simulink model "PM_Motor_Ver2015"  (R2015a)
settings: Solver=VariableStepDiscrete  StartTime=0.0  StopTime=1  RelTol=1e-3
PreLoadFcn:
  | Ts=5e-6;
undefined symbols (not defined in the file): ctrl_sat, pos_Kp, Pos_Target, speed_Ki, speed_Kp, Speed_Target
libraries: powerlib x16, powerlib_extras x3, simulink x1, AC6DriveInternalModels x1
settings Model: ExtModeAutoUpdateStatusClock=off  Creator=batserve  LastModifiedBy=Savvas
settings DataIOCC: SignalLoggingSaveFormat=ModelDataLogs  SaveOutput=off  SignalLogging=off  SaveTime=off  SignalLoggingName=sigsOut
settings OptimizationCC: ExpressionDepthLimit=2147483647  InitFltsAndDblsToZero=on
settings DebuggingCC: SaveWithParameterizedLinksMsg=none  UnderspecifiedInitializationDetection=Classic  MergeDetectMultiDrivingBlocksExec=none  CheckExecutionContextPreStartOutputMsg=on  CheckExecutionContextRuntimeOutputMsg=on  SignalResolutionControl=TryResolveAllWithWarning  MultiTaskDSMMsg=warning  MultiTaskCondExecSysMsg=none  FcnCallInpInsideContextMsg=UseLocalSettings  StateNameClashWarn=warning
settings HardwareCC: TargetUnknown=on
settings GRTTargetCC: TargetFcnLib=ansi_tfl_tmw.mat  CombineOutputUpdateFcns=off  GRTInterface=on

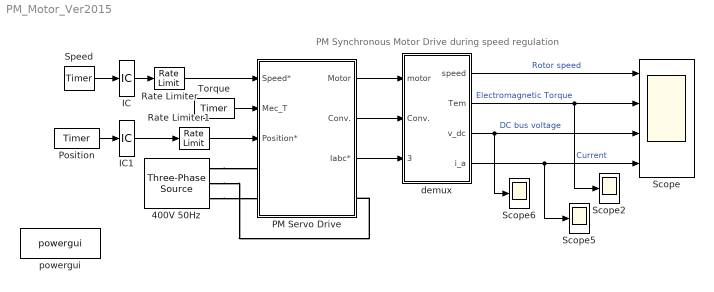
== system PM_Motor_Ver2015 ==
  note: PM Synchronous Motor Drive during speed regulation
  400V 50Hz : powerlib/Electrical Sources/Three-Phase Source  Voltage=400  PhaseAngle=0  Frequency=60  InternalConnection=Yg  SpecifyImpedance=off  Resistance=0.02  Inductance=0.05e-3  ShortCircuitLevel=100e6  BaseVoltage=25e3  XRratio=7  BusType=swing  Pref=0  Qref=0  Qmin=-inf  Qmax=inf
  IC : InitialCondition  Value=0
  IC1 : InitialCondition  Value=0
  PM Servo Drive : Subsystem
  Position : powerlib_extras/Control  Blocks/Timer  t=[0 1]  e=[1 1]*Pos_Target
  Rate Limiter : RateLimiter  RisingSlewLimit=600000  FallingSlewLimit=-600000  LinearizeAsGain=off
  Rate Limiter1 : RateLimiter  RisingSlewLimit=2000  FallingSlewLimit=-2000  SampleTimeMode=inherited  LinearizeAsGain=off
  Scope : Scope  NumInputPorts=4
      settings: TimeRange=0.5  YMin=-1500~-30~0~-60  YMax=1500~30~1000~60  SaveName=simout
  Scope2 : Scope
      settings: YMin=-15  YMax=25  SaveName=Torque
  Scope5 : Scope
      settings: TimeRange=0.06746987951807232  YMin=-30.19796761679877  YMax=24.82817507168159  SaveName=Current
  Scope6 : Scope
      settings: YMin=-1500  YMax=1500  SaveName=DC_voltage
  Speed : powerlib_extras/Control  Blocks/Timer  t=[0 1]  e=[1 1]*Speed_Target
  Torque : powerlib_extras/Control  Blocks/Timer  t=Mech_Load_Time  e=Mech_Load
  demux : Subsystem
  powergui : powerlib/powergui  Priority=2  SimulationMode=Discrete  SolverType=Tustin  SampleTime=Ts  frequency=60  SPID=off  DisableSnubberDevices=off  DisableRonSwitches=off  DisableVfSwitches=off  SwTol=0  DisplayEquations=off  Interpol=off  methode=off  Ts=0  FunctionMessages=off  echomessages=off  HookPort=off  EnableUseOfTLC=off  x0status=blocks  frequencyindice=60  Pbase=100e6  ErrMax=1e-4  Iterations=50  UnitsV=kV  UnitsW=MW  buscounter=0  RestoreLinks=warning  ResistiveCurrentMeasurement=off  Frange=[0:2:500]  Ylog=off  Xlog=on  ShowGrid=off  save=off  variable=ZData  structure=0  ZoomFFT=on  StartTime=0.0  cycles=1  DisplayStyle=1  fundamental=60  FreqAxis=off  MaxFrequency=1000  frequencyindicesteady=1  RmsSteady=1  display=off
  wires:
  Torque/1 -> PM Servo Drive/2(Mec_T)
  PM Servo Drive/1(Motor) -> demux/1(motor)
  PM Servo Drive/2(Conv.) -> demux/2(Conv.)
  PM Servo Drive/3(Iabc*) -> demux/3(Conv.2)
  demux/1(speed) -> Scope/1  "Rotor speed"
  demux/2(Tem) -> Scope/2, Scope2/1  "Electromagnetic Torque"
  demux/3(v_dc) -> Scope/3, Scope6/1  "DC bus voltage"
  demux/4(i_a) -> Scope/4, Scope5/1  "Current"
  Speed/1 -> IC/1
  Position/1 -> IC1/1
  Rate Limiter/1 -> PM Servo Drive/1(Speed*)
  Rate Limiter1/1 -> PM Servo Drive/3(Position*)
  IC/1 -> Rate Limiter/1
  IC1/1 -> Rate Limiter1/1
  connections:
  400V 50Hz/RConn1 -- PM Servo Drive/LConn1
  400V 50Hz/RConn2 -- PM Servo Drive/RConn1
  400V 50Hz/RConn3 -- PM Servo Drive/LConn2

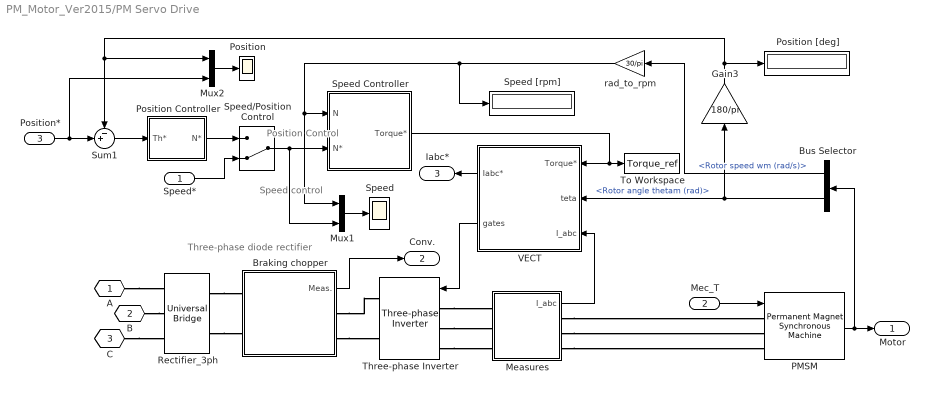
== system PM_Motor_Ver2015/PM Servo Drive ==
  note: Three-phase
      | diode rectifier
  note: Speed
      | control
  note: Position
      |  Control
  Speed* : Inport
  Mec_T : Inport  Port=2
  Position* : Inport  Port=3
  Braking chopper : Subsystem  mask(Braking chopper){chopa=650, chopd=530, freq_chop=1000, cap_bus=1500e-6, br=30}
      mask prompts: chopa "Chopper activation voltage (V)"; chopd "Chopper shutdown voltage (V)"; freq_chop "Braking chopper frequency (Hz)"; cap_bus "DC bus capacitance (F)"; br "Braking resistance (ohms)"
      mask help: This block implements a DC link between the rectifier and the inverter. It also contains a DC bus integrated braking chopper. The braking resistor must be set properly to avoid oscillation.
      mask init:
      | [X1,X1m,X2,X2m,X3,X4,Y1,Y1m,Y2,Y2m,Y3,Y4,color1,color2]=spsdrivelogo;
      mask Display:
      | patch([X1 X1m],[Y1 Y1m],color1);
      | patch(X3,Y3,color2);
      | plot([X1 X1m X2 X2m X3 X4],[Y1 Y1m Y2 Y2m Y3 Y4]);
  Bus Selector : BusSelector  OutputSignals=Rotor speed wm (rad/s),Rotor angle thetam (rad)
  Gain3 : Gain  Gain=180/pi  SampleTime=1e-3  SaturateOnIntegerOverflow=on  OutDataTypeStr=Inherit: Same as input  ParamDataTypeStr=Inherit: Same as input
  Measures : Subsystem
  Mux1 : Mux  Inputs=2
  Mux2 : Mux  Inputs=2
  PMSM : powerlib/Machines/Permanent Magnet Synchronous Machine  NbPhases=3  FluxDistribution=Sinusoidal  RotorType=Round  MechanicalLoad=Torque Tm  PresetModel=No  ShowDetailedParameters=on  MeasurementBus=off  Resistance=2.1  Inductance=8.5e-3  dqInductances=[0.015 0.015]  La=0.009  MachineConstant=Flux linkage established by magnets (V.s)  Flux=0.22  VoltageCst=159.6143  TorqueCst=1.32  Flat=120  Mechanical=[0.028 0 4]  PolePairs=4  InitialConditions=[0,0, 0,0]  InitialConditions5ph=[0 0 0 0 0 0]  TsPowergui=0  TsBlock=-1  RefAngle=90 degrees behind phase A axis (modified Park)
  Position : Scope
      settings: YMin=-50  YMax=700  SaveName=Rotor_angle1
  Position Controller : Subsystem  mask{Kp_th=pos_Kp, T_position=5e-3}
      mask prompts: Kp_th "Proportional gain"; T_position "Controllersampling time (s)"
  Position [deg] : Display
  Rectifier_3ph : powerlib/Power Electronics/Universal Bridge  Arms=3  SnubberResistance=10e3  SnubberCapacitance=20e-9  Device=Diodes  Ron=1e-3  Lon=0  ForwardVoltages="[  0,  0  ]"  ForwardVoltage=1.3  GTOparameters=[ 10e-6, 20e-6 ]  IGBTparameters=[ 1e-6 , 2e-6 ]  Measurements=All voltages and currents  Measurements_2=None  converterType=Rectifier
  Speed : Scope
      settings: YMin=-100  YMax=1300  SaveName=speed_ref1
  Speed Controller : Subsystem  mask(Speed controller){kp=speed_Kp, ki=speed_Ki, fc=30, ctrl_sat=[-25,25], Tsc=5e-3}
      mask prompts: kp "Proportional gain"; ki "Integral gain"; fc "Speed measurement - low-pass filter cutoff frequency (Hz)"; ctrl_sat "Controller output torque saturation (N.m) [negative,positive]"; Tsc "Controller sampling time (s)"
      mask help: This block implements a PI speed regulator.
      mask init:
      | [X1,X1m,X2,X2m,X3,X4,Y1,Y1m,Y2,Y2m,Y3,Y4,color1,color2]=spsdrivelogo;
      mask Display:
      | patch([X1 X1m],[Y1 Y1m],color1);
      | patch(X3,Y3,color2);
      | plot([X1 X1m X2 X2m X3 X4],[Y1 Y1m Y2 Y2m Y3 Y4]);
  Speed [rpm] : Display
  Speed/Position Control : ManualSwitch  CurrentSetting=0
  Sum1 : Sum  Inputs=-+|  SaturateOnIntegerOverflow=on  InputSameDT=on  OutDataTypeStr=Inherit: Same as first input
  Three-phase Inverter : AC6DriveInternalModels/Three-phase Inverter  Arms=3  SnubberResistance=5000  SnubberCapacitance=inf  Device=IGBT / Diodes  Ron=1e-3  Lon=0  ForwardVoltages=[0.8,0.8]  ForwardVoltage=0  GTOparameters=[0,0]  IGBTParameters=[1e-6,2e-6]  Measurements=All voltages and currents  converterType=Inverter  SourceFrequency=60  dqInductances=[8.5e-3,8.5e-3]  Flux=0.175  Resistance=0.2  p=4
  To Workspace : ToWorkspace  VariableName=Torque_ref  SampleTime=-1
      settings: Save2DSignal=2-D array (concatenate along first dimension)
  VECT : Subsystem  AncestorBlock=AC6DriveInternalModels/VECT  mask(VECT){nb_p=4, lambda=0.22, Id=0, Rs=2.1, Ld=0.009, freq_max=20e3, Ts_vect=50e-6}
      mask prompts: nb_p "Motor pairs of poles"; lambda "Flux induced by magnets (Wb)"; Id "d-axis current, Id (A)"; Rs "Stator resistance (Ohm)"; Ld "Inductanse (Ld=Lq), [H]"; freq_max "Maximum switching frequency (Hz)"; Ts_vect "Sampling time (s)"
      mask help: This block implements a vector controller.
      mask init:
      | [X1,X1m,X2,X2m,X3,X4,Y1,Y1m,Y2,Y2m,Y3,Y4,color1,color2]=spsdrivelogo;
      mask Display:
      | patch([X1 X1m],[Y1 Y1m],color1);
      | patch(X3,Y3,color2);
      | plot([X1 X1m X2 X2m X3 X4],[Y1 Y1m Y2 Y2m Y3 Y4]);
  rad_to_rpm : Gain  Gain=30/pi  SampleTime=1e-3  SaturateOnIntegerOverflow=on  OutDataTypeStr=Inherit: Same as input  ParamDataTypeStr=Inherit: Same as input
  A : PMIOPort  Port=1  Side=Left
  B : PMIOPort  Port=2  Side=Right
  C : PMIOPort  Tag=PMCPort  Port=3  Side=Left
  Motor : Outport
  Conv. : Outport  Port=2
  Iabc* : Outport  Port=3
  wires:
  Bus Selector/2 -> Gain3/1, VECT/2(teta)  "<Rotor angle thetam (rad)>"
  Bus Selector/1 -> rad_to_rpm/1  "<Rotor speed wm (rad/s)>"
  VECT/2(gates) -> Three-phase Inverter/1
  Speed Controller/1(Torque*) -> To Workspace/1, VECT/1(Torque*)
  Measures/1(I_abc) -> VECT/3(I_abc)
  PMSM/1 -> Motor/1, Bus Selector/1
  Braking chopper/1(Meas.) -> Conv./1
  VECT/1(Iabc*) -> Iabc*/1
  Gain3/1 -> Sum1/1, Mux2/1, Position [deg]/1
  Position*/1 -> Sum1/2, Mux2/2
  Sum1/1 -> Position Controller/1(Th*)
  Mux2/1 -> Position/1
  Speed/Position Control/1 -> Speed Controller/2(N*), Mux1/2
  Position Controller/1(N*) -> Speed/Position Control/1
  Speed*/1 -> Speed/Position Control/2
  Mux1/1 -> Speed/1
  rad_to_rpm/1 -> Speed Controller/1(N), Mux1/1, Speed [rpm]/1
  Mec_T/1 -> PMSM/1
  connections:
  Rectifier_3ph/RConn2 -- Braking chopper/LConn2
  Rectifier_3ph/RConn1 -- Braking chopper/LConn1
  Three-phase Inverter/LConn2 -- Measures/LConn2
  Braking chopper/RConn1 -- Three-phase Inverter/RConn1
  Braking chopper/RConn2 -- Three-phase Inverter/RConn2
  A/RConn1 -- Rectifier_3ph/LConn1
  Measures/RConn1 -- PMSM/LConn1
  Measures/RConn2 -- PMSM/LConn2
  B/RConn1 -- Rectifier_3ph/LConn2
  Three-phase Inverter/LConn3 -- Measures/LConn3
  Measures/RConn3 -- PMSM/LConn3
  C/RConn1 -- Rectifier_3ph/LConn3
  Three-phase Inverter/LConn1 -- Measures/LConn1

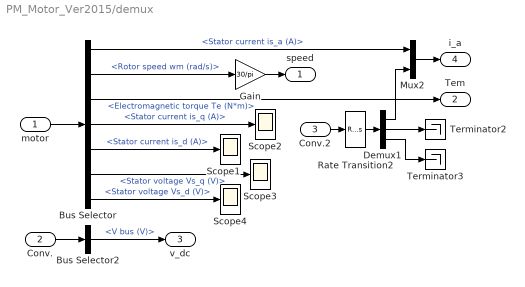
== system PM_Motor_Ver2015/demux ==
  motor : Inport
  Conv. : Inport  Port=2
  Conv.2 : Inport  Port=3
  Bus Selector : BusSelector  OutputSignals=Stator current is_a (A),Rotor speed wm (rad/s),Electromagnetic torque Te (N*m),Stator current is_q (A),Stator current is_d (A),Stator voltage Vs_q (V),Stator voltage Vs_d (V)
  Bus Selector2 : BusSelector  OutputSignals=V bus (V)
  Demux1 : Demux  Outputs=3
  Gain : Gain  Gain=30/pi  SaturateOnIntegerOverflow=on  OutDataTypeStr=Inherit: Same as input  ParamDataTypeStr=Inherit: Same as input
  Mux2 : Mux  Inputs=2
  Rate Transition2 : RateTransition
  Scope{1..4} (4 alike) : Scope
      Scope1 settings: YMin=-10  YMax=10  SaveName=Id
      Scope2 settings: YMin=15.5  YMax=22  SaveName=Iq
      Scope3 settings: YMin=5.6  YMax=6.7  SaveName=Vsq
      Scope4 settings: YMin=5.6  YMax=6.7  SaveName=Vsd
  Terminator2 : Terminator
  Terminator3 : Terminator
  speed : Outport
  Tem : Outport  Port=2
  v_dc : Outport  Port=3
  i_a : Outport  Port=4
  wires:
  Bus Selector/2 -> Gain/1  "<Rotor speed wm (rad/s)>"
  Bus Selector2/1 -> v_dc/1  "<V bus (V)>"
  Conv./1 -> Bus Selector2/1
  Gain/1 -> speed/1
  Bus Selector/1 -> Mux2/1  "<Stator current is_a (A)>"
  Bus Selector/3 -> Tem/1  "<Electromagnetic torque Te (N*m)>"
  motor/1 -> Bus Selector/1
  Mux2/1 -> i_a/1
  Conv.2/1 -> Rate Transition2/1
  Rate Transition2/1 -> Demux1/1
  Demux1/1 -> Mux2/2
  Bus Selector/4 -> Scope2/1  "<Stator current is_q (A)>"
  Bus Selector/5 -> Scope1/1  "<Stator current is_d (A)>"
  Bus Selector/6 -> Scope3/1  "<Stator voltage Vs_q (V)>"
  Bus Selector/7 -> Scope4/1  "<Stator voltage Vs_d (V)>"
  Demux1/3 -> Terminator3/1
  Demux1/2 -> Terminator2/1

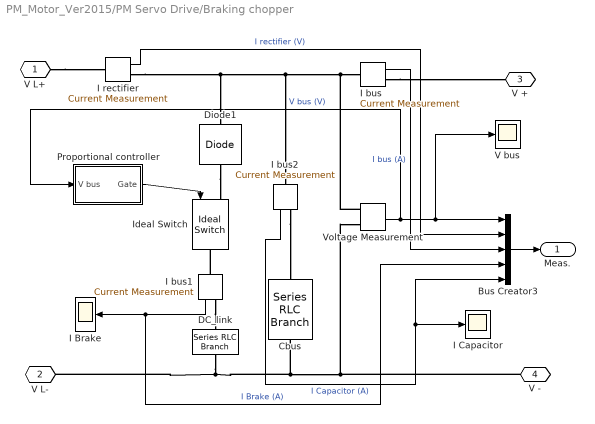
== system PM_Motor_Ver2015/PM Servo Drive/Braking chopper ==
  Bus Creator3 : BusCreator  Inputs=5
  Cbus : powerlib/Elements/Series RLC Branch  LConnTagsString=__new0  RConnTagsString=__new0  BranchType=C  Resistance=[]  Inductance=[]  SetiL0=off  InitialCurrent=0  Capacitance=cap_bus  Setx0=off  InitialVoltage=0  Measurements=None
  DC_link : powerlib/Elements/Series RLC Branch  LConnTagsString=__new0  RConnTagsString=__new0  BranchType=R  Resistance=br  Inductance=[]  SetiL0=off  InitialCurrent=0  Capacitance=[]  Setx0=off  InitialVoltage=0  Measurements=None
  Diode1 : powerlib/Power Electronics/Diode  Ron=0.01  Lon=0  Vf=0.8  IC=0  UseSnubber=off  Rs=10  Cs=10e-9  Measurements=off
  I Brake : Scope
      settings: YMin=-2.5  YMax=32.5  SaveName=simout2  Decimation=25
  I Capacitor : Scope
      settings: TimeRange=2  YMin=-200  YMax=200  SaveName=simout4
  I bus : powerlib/Measurements/Current Measurement  PhasorSimulation=off  OutputType=Complex  PSBequivalent=0
  I bus1 : powerlib/Measurements/Current Measurement  PhasorSimulation=off  OutputType=Complex  PSBequivalent=0
  I bus2 : powerlib/Measurements/Current Measurement  PhasorSimulation=off  OutputType=Complex  PSBequivalent=0
  I rectifier : powerlib/Measurements/Current Measurement  PhasorSimulation=off  OutputType=Complex  PSBequivalent=0
  Ideal Switch : powerlib/Power Electronics/Ideal Switch  Ron=0.01  Lon=0  IC=0  Rs=0.1  Cs=0.01e-6  Measurements=off
      settings: AttributesFormatString=\n
  Proportional controller : Subsystem
  V bus : Scope
      settings: TimeRange=2  YMin=0  YMax=950  SaveName=simout5
  Voltage Measurement : powerlib/Measurements/Voltage Measurement  Tag=PoWeRsYsTeMmEaSuReMeNt  PhasorSimulation=off  OutputType=Complex  PSBequivalent=0
  V L+ : PMIOPort  Port=1  Side=Left
  V L- : PMIOPort  Port=2  Side=Left
  V + : PMIOPort  Port=3  Side=Right
  V - : PMIOPort  Port=4  Side=Right
  Meas. : Outport
  wires:
  Voltage Measurement/1 -> Bus Creator3/1, V bus/1, Proportional controller/1(V bus)  "V bus (V)"
  Proportional controller/1(Gate) -> Ideal Switch/1
  Bus Creator3/1 -> Meas./1
  I bus/1 -> Bus Creator3/3  "I bus (A)"
  I rectifier/1 -> Bus Creator3/2  "I rectifier (V)"
  I bus1/1 -> I Brake/1, Bus Creator3/4  "I Brake (A)"
  I bus2/1 -> Bus Creator3/5, I Capacitor/1  "I Capacitor (A)"
  connections:
  Cbus/RConn1 -- V -/RConn1 -- Voltage Measurement/LConn2 -- V L-/RConn1 -- DC_link/RConn1
  Diode1/LConn1 -- I rectifier/RConn1 -- Voltage Measurement/LConn1 -- I bus/LConn1 -- I bus2/LConn1
  Diode1/RConn1 -- Ideal Switch/LConn1
  I bus/RConn1 -- V +/RConn1
  V L+/RConn1 -- I rectifier/LConn1
  I bus1/RConn1 -- DC_link/LConn1
  I bus1/LConn1 -- Ideal Switch/RConn1
  I bus2/RConn1 -- Cbus/LConn1

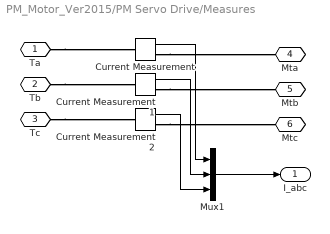
== system PM_Motor_Ver2015/PM Servo Drive/Measures ==
  Current Measurement : powerlib/Measurements/Current Measurement  Tag=PoWeRsYsTeMmEaSuReMeNt  PhasorSimulation=off  OutputType=Magnitude  PSBequivalent=0
  Current Measurement1 : powerlib/Measurements/Current Measurement  Tag=PoWeRsYsTeMmEaSuReMeNt  PhasorSimulation=off  OutputType=Magnitude  PSBequivalent=0
  Current Measurement2 : powerlib/Measurements/Current Measurement  Tag=PoWeRsYsTeMmEaSuReMeNt  PhasorSimulation=off  OutputType=Magnitude  PSBequivalent=0
  Mux1 : Mux  Inputs=3
  Ta : PMIOPort  Port=1  Side=Left
  Tb : PMIOPort  Port=2  Side=Left
  Tc : PMIOPort  Port=3  Side=Left
  Mta : PMIOPort  Port=4  Side=Right
  Mtb : PMIOPort  Port=5  Side=Right
  Mtc : PMIOPort  Port=6  Side=Right
  I_abc : Outport
  wires:
  Current Measurement1/1 -> Mux1/2
  Current Measurement/1 -> Mux1/1
  Current Measurement2/1 -> Mux1/3
  Mux1/1 -> I_abc/1
  connections:
  Current Measurement1/RConn1 -- Mtb/RConn1
  Tb/RConn1 -- Current Measurement1/LConn1
  Current Measurement/RConn1 -- Mta/RConn1
  Ta/RConn1 -- Current Measurement/LConn1
  Tc/RConn1 -- Current Measurement2/LConn1
  Current Measurement2/RConn1 -- Mtc/RConn1

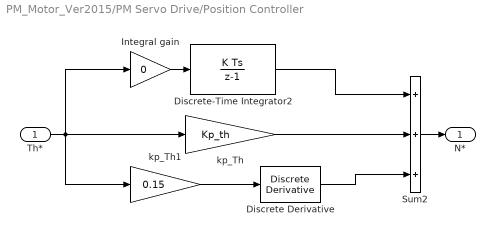
== system PM_Motor_Ver2015/PM Servo Drive/Position Controller ==
  Th* : Inport
  Discrete Derivative : simulink/Discrete/Discrete Derivative  gainval=1.0  ICPrevScaledInput=0.0  InputProcessing=Inherited  OutMin=[]  OutMax=[]  OutDataType=fixdt(1, 16)  OutScaling=2^-10  DoSatur=off
  Discrete-Time Integrator2 : DiscreteIntegrator  SampleTime=-1  UpperSaturationLimit=ctrl_sat(2)/3  LowerSaturationLimit=ctrl_sat(1)/3
  Integral gain : Gain  Gain=0  SampleTime=T_position  SaturateOnIntegerOverflow=on  OutDataTypeStr=Inherit: Same as input  ParamDataTypeStr=Inherit: Same as input
  Sum2 : Sum  Inputs=+++  SaturateOnIntegerOverflow=on  InputSameDT=on  OutDataTypeStr=Inherit: Same as first input
  kp_Th : Gain  Gain=Kp_th  SampleTime=T_position  SaturateOnIntegerOverflow=on  OutDataTypeStr=Inherit: Same as input  ParamDataTypeStr=Inherit: Same as input
  kp_Th1 : Gain  Gain=0.15  SampleTime=T_position  SaturateOnIntegerOverflow=on  OutDataTypeStr=Inherit: Same as input  ParamDataTypeStr=Inherit: Same as input
  N* : Outport
  wires:
  Th*/1 -> kp_Th/1, Integral gain/1, kp_Th1/1
  Sum2/1 -> N*/1
  Integral gain/1 -> Discrete-Time Integrator2/1
  Discrete Derivative/1 -> Sum2/3
  kp_Th/1 -> Sum2/2
  Discrete-Time Integrator2/1 -> Sum2/1
  kp_Th1/1 -> Discrete Derivative/1

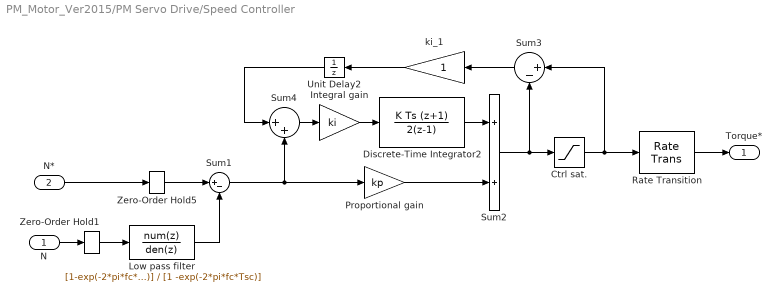
== system PM_Motor_Ver2015/PM Servo Drive/Speed Controller ==
  N : Inport
  N* : Inport  Port=2
  Ctrl sat. : Saturate  UpperLimit=ctrl_sat(2)  LowerLimit=ctrl_sat(1)
  Discrete-Time Integrator2 : DiscreteIntegrator  IntegratorMethod=Integration: Trapezoidal  SampleTime=Tsc  LimitOutput=on  UpperSaturationLimit=ctrl_sat(2)/3  LowerSaturationLimit=ctrl_sat(1)/3
  Integral gain : Gain  Gain=ki  SampleTime=Tsc  SaturateOnIntegerOverflow=on  OutDataTypeStr=Inherit: Same as input  ParamDataTypeStr=Inherit: Same as input
  Low pass filter : DiscreteTransferFcn  Numerator=[1-exp(-2*pi*fc*Tsc)]  Denominator=[1 -exp(-2*pi*fc*Tsc)]  SampleTime=Tsc
  Proportional gain : Gain  Gain=kp  SampleTime=Tsc  SaturateOnIntegerOverflow=on  OutDataTypeStr=Inherit: Same as input  ParamDataTypeStr=Inherit: Same as input
  Rate Transition : RateTransition
  Sum1 : Sum  Inputs=|+-  SaturateOnIntegerOverflow=on  InputSameDT=on  OutDataTypeStr=Inherit: Same as first input
  Sum2 : Sum  SaturateOnIntegerOverflow=on  InputSameDT=on  OutDataTypeStr=Inherit: Same as first input
  Sum3 : Sum  Inputs=|+-
  Sum4 : Sum  Inputs=|++
  Unit Delay2 : UnitDelay  SampleTime=-1
  Zero-Order Hold1 : ZeroOrderHold  SampleTime=Tsc
  Zero-Order Hold5 : ZeroOrderHold  SampleTime=Tsc
  ki_1 : Gain  SaturateOnIntegerOverflow=on  OutDataTypeStr=Inherit: Same as input  ParamDataTypeStr=Inherit: Same as input
  Torque* : Outport
  wires:
  N*/1 -> Zero-Order Hold5/1
  Ctrl sat./1 -> Sum3/1, Rate Transition/1
  N/1 -> Zero-Order Hold1/1
  Rate Transition/1 -> Torque*/1
  Zero-Order Hold1/1 -> Low pass filter/1
  Zero-Order Hold5/1 -> Sum1/1
  Sum2/1 -> Ctrl sat./1, Sum3/2
  Sum1/1 -> Proportional gain/1, Sum4/2
  Low pass filter/1 -> Sum1/2
  Integral gain/1 -> Discrete-Time Integrator2/1
  Sum3/1 -> ki_1/1
  ki_1/1 -> Unit Delay2/1
  Discrete-Time Integrator2/1 -> Sum2/1
  Proportional gain/1 -> Sum2/2
  Sum4/1 -> Integral gain/1
  Unit Delay2/1 -> Sum4/1

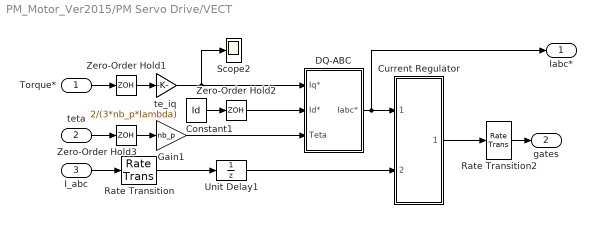
== system PM_Motor_Ver2015/PM Servo Drive/VECT ==
  Torque* : Inport
  teta : Inport  Port=2
  I_abc : Inport  Port=3
  Constant1 : Constant  Value=Id
  Current Regulator : Subsystem
  DQ-ABC : Subsystem
  Gain1 : Gain  Gain=nb_p  SaturateOnIntegerOverflow=on  OutDataTypeStr=Inherit: Same as input  ParamDataTypeStr=Inherit: Same as input
  Rate Transition : RateTransition
  Rate Transition2 : RateTransition
  Scope2 : Scope
      settings: YMin=22.75  YMax=24.5  SaveName=Iq_Ref
  Unit Delay1 : UnitDelay  SampleTime=Ts_vect
  Zero-Order Hold1 : ZeroOrderHold  SampleTime=Ts_vect
  Zero-Order Hold2 : ZeroOrderHold  SampleTime=Ts_vect
  Zero-Order Hold3 : ZeroOrderHold  SampleTime=Ts_vect
  te_iq : Gain  Gain=2/(3*nb_p*lambda)  SaturateOnIntegerOverflow=on  OutDataTypeStr=Inherit: Same as input  ParamDataTypeStr=Inherit: Same as input
  Iabc* : Outport
  gates : Outport  Port=2
  wires:
  Zero-Order Hold2/1 -> DQ-ABC/2("Id* ")
  Rate Transition/1 -> Unit Delay1/1
  Zero-Order Hold1/1 -> te_iq/1
  teta/1 -> Zero-Order Hold3/1
  Zero-Order Hold3/1 -> Gain1/1
  Torque*/1 -> Zero-Order Hold1/1
  Constant1/1 -> Zero-Order Hold2/1
  Gain1/1 -> DQ-ABC/3(Teta)
  Unit Delay1/1 -> Current Regulator/2(Iabc)
  DQ-ABC/1(Iabc*) -> Current Regulator/1(Iabc*), Iabc*/1
  I_abc/1 -> Rate Transition/1
  te_iq/1 -> Scope2/1, DQ-ABC/1("Iq* ")
  Current Regulator/1(Pulses) -> Rate Transition2/1
  Rate Transition2/1 -> gates/1

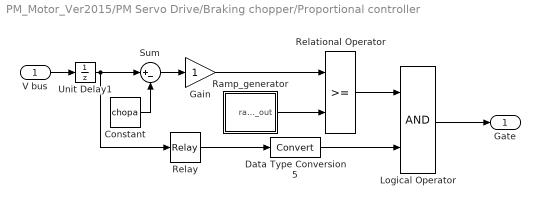
== system PM_Motor_Ver2015/PM Servo Drive/Braking chopper/Proportional controller ==
  V bus : Inport
  Constant : Constant  Value=chopa
  Data Type Conversion5 : DataTypeConversion  SaturateOnIntegerOverflow=on  RndMeth=Zero
  Gain : Gain  SaturateOnIntegerOverflow=on  OutDataTypeStr=Inherit: Same as input  ParamDataTypeStr=Inherit: Same as input
  Logical Operator : Logic
  Ramp_generator : Subsystem
  Relational Operator : RelationalOperator  InputSameDT=on
  Relay : Relay  OnSwitchValue=chopa  OffSwitchValue=chopd
  Sum : Sum  Inputs=|+-  SaturateOnIntegerOverflow=on  InputSameDT=on  OutDataTypeStr=Inherit: Same as first input
  Unit Delay1 : UnitDelay  SampleTime=Ts
  Gate : Outport
  wires:
  Data Type Conversion5/1 -> Logical Operator/2
  Relay/1 -> Data Type Conversion5/1
  Logical Operator/1 -> Gate/1
  Relational Operator/1 -> Logical Operator/1
  V bus/1 -> Unit Delay1/1
  Constant/1 -> Sum/2
  Gain/1 -> Relational Operator/1
  Sum/1 -> Gain/1
  Unit Delay1/1 -> Relay/1, Sum/1
  Ramp_generator/1(ramp_out) -> Relational Operator/2

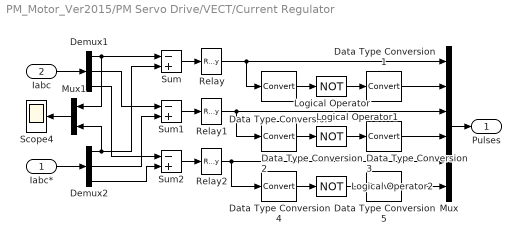
== system PM_Motor_Ver2015/PM Servo Drive/VECT/Current Regulator ==
  Iabc* : Inport
  Iabc : Inport  Port=2
  Data Type Conversion{,1..5} (6 alike) : DataTypeConversion  SaturateOnIntegerOverflow=on  RndMeth=Zero
  Demux1 : Demux  Outputs=3
  Demux2 : Demux  Outputs=3
  Logical Operator : Logic  Operator=NOT
  Logical Operator1 : Logic  Operator=NOT
  Logical Operator2 : Logic  Operator=NOT
  Mux : Mux  Inputs=6
  Mux1 : Mux  Inputs=2
  Relay : Relay  OnSwitchValue=0  OffSwitchValue=0
  Relay1 : Relay  OnSwitchValue=0  OffSwitchValue=0
  Relay2 : Relay  OnSwitchValue=0  OffSwitchValue=0
  Scope4 : Scope
      settings: TimeRange=0.06  YMin=-30  YMax=30  SaveName=Ia_ref
  Sum : Sum  Inputs=-+  SaturateOnIntegerOverflow=on  InputSameDT=on  OutDataTypeStr=Inherit: Same as first input
  Sum1 : Sum  Inputs=-+  SaturateOnIntegerOverflow=on  InputSameDT=on  OutDataTypeStr=Inherit: Same as first input
  Sum2 : Sum  Inputs=-+  SaturateOnIntegerOverflow=on  InputSameDT=on  OutDataTypeStr=Inherit: Same as first input
  Pulses : Outport  InitialOutput=0
  wires:
  Data Type Conversion5/1 -> Mux/6
  Data Type Conversion4/1 -> Logical Operator2/1
  Data Type Conversion3/1 -> Mux/4
  Data Type Conversion2/1 -> Logical Operator1/1
  Data Type Conversion1/1 -> Mux/2
  Data Type Conversion/1 -> Logical Operator/1
  Sum/1 -> Relay/1
  Sum1/1 -> Relay1/1
  Demux1/1 -> Sum/1, Mux1/1
  Demux1/2 -> Sum1/1
  Mux/1 -> Pulses/1
  Iabc/1 -> Demux1/1
  Sum2/1 -> Relay2/1
  Demux1/3 -> Sum2/1
  Demux2/3 -> Sum2/2
  Demux2/2 -> Sum1/2
  Demux2/1 -> Sum/2, Mux1/2
  Iabc*/1 -> Demux2/1
  Relay/1 -> Data Type Conversion/1, Mux/1
  Relay1/1 -> Data Type Conversion2/1, Mux/3
  Relay2/1 -> Data Type Conversion4/1, Mux/5
  Logical Operator/1 -> Data Type Conversion1/1
  Logical Operator1/1 -> Data Type Conversion3/1
  Logical Operator2/1 -> Data Type Conversion5/1
  Mux1/1 -> Scope4/1

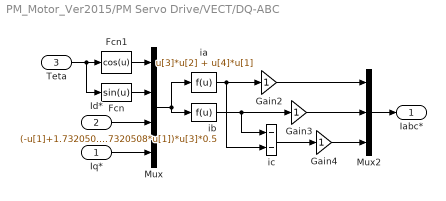
== system PM_Motor_Ver2015/PM Servo Drive/VECT/DQ-ABC ==
  "Iq* " : Inport
  "Id* " : Inport  Port=2
  Teta : Inport  Port=3
  Fcn : Fcn  Expr=sin(u)
  Fcn1 : Fcn  Expr=cos(u)
  Gain2 : Gain  SaturateOnIntegerOverflow=on  OutDataTypeStr=Inherit: Same as input  ParamDataTypeStr=Inherit: Same as input
  Gain3 : Gain  SaturateOnIntegerOverflow=on  OutDataTypeStr=Inherit: Same as input  ParamDataTypeStr=Inherit: Same as input
  Gain4 : Gain  SaturateOnIntegerOverflow=on  OutDataTypeStr=Inherit: Same as input  ParamDataTypeStr=Inherit: Same as input
  Mux : Mux
  Mux2 : Mux  Inputs=3
  ia : Fcn  Expr=u[3]*u[2] + u[4]*u[1]
  ib : Fcn  Expr=(-u[1]+1.7320508*u[2])*u[4]*0.5-(u[2]+1.7320508*u[1])*u[3]*0.5
  ic : Sum  Inputs=--  SaturateOnIntegerOverflow=on  InputSameDT=on  OutDataTypeStr=Inherit: Same as first input
  Iabc* : Outport  InitialOutput=0
  wires:
  Fcn/1 -> Mux/2
  Fcn1/1 -> Mux/1
  Mux2/1 -> Iabc*/1
  Mux/1 -> ib/1, ia/1
  Teta/1 -> Fcn1/1, Fcn/1
  "Id* "/1 -> Mux/3
  "Iq* "/1 -> Mux/4
  Gain3/1 -> Mux2/2
  ic/1 -> Gain4/1
  Gain4/1 -> Mux2/3
  Gain2/1 -> Mux2/1
  ia/1 -> Gain2/1, ic/2
  ib/1 -> Gain3/1, ic/1

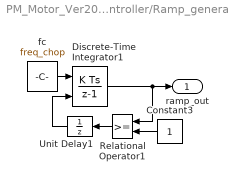
== system PM_Motor_Ver2015/PM Servo Drive/Braking chopper/Proportional controller/Ramp_generator ==
  Constant3 : Constant
  Discrete-Time Integrator1 : DiscreteIntegrator  ExternalReset=rising  SampleTime=Ts
  Relational Operator1 : RelationalOperator  InputSameDT=on
  Unit Delay1 : UnitDelay  SampleTime=Ts
  fc : Constant  Value=freq_chop
  ramp_out : Outport
  wires:
  Unit Delay1/1 -> Discrete-Time Integrator1/2
  Relational Operator1/1 -> Unit Delay1/1
  Constant3/1 -> Relational Operator1/2
  Discrete-Time Integrator1/1 -> ramp_out/1, Relational Operator1/1
  fc/1 -> Discrete-Time Integrator1/1
